simulink model "PMSM_FOC_Component_Baseline"  (R2025b)
settings: Solver=FixedStepDiscrete  StartTime=0.0  StopTime=4  FixedStep=0.0001  RelTol=1e-3
settings Model: Creator=Wu  LastModifiedBy=Wu
settings DataIOCC: SaveFormat=StructureWithTime  SignalLogging=off

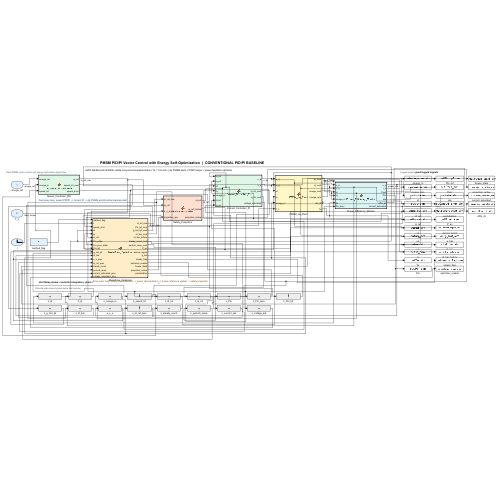
[thumbnail: Simulink's stored preview of the top-level diagram]
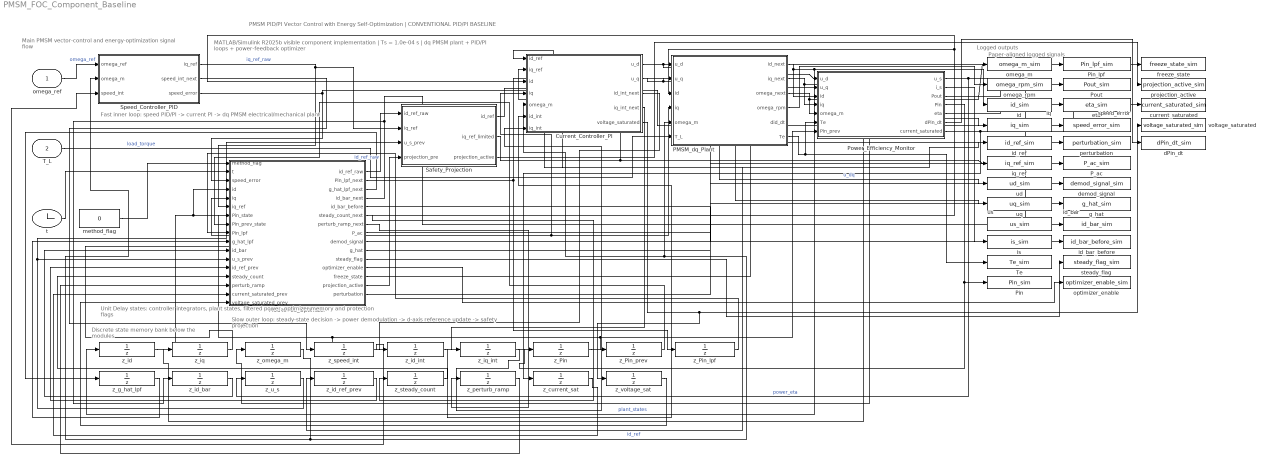
== system PMSM_FOC_Component_Baseline ==
  note: Main PMSM vector-control and energy-optimization signal flow
  note: Discrete state memory bank below the modules
  note: Logged outputs
  note: PMSM PID/PI Vector Control with Energy Self-Optimization | CONVENTIONAL PID/PI BASELINE
  note: MATLAB/Simulink R2025b visible component implementation | Ts = 1.0e-04 s | dq PMSM plant + PID/PI loops + power-feedback optimizer
  note: Fast inner loop: speed PID/PI -> current PI -> dq PMSM electrical/mechanical plant
  note: Slow outer loop: steady-state decision -> power demodulation -> d-axis reference update -> safety projection
  note: Unit Delay states: controller integrators, plant states, filtered power, optimizer memory and protection flags
  note: Paper-aligned logged signals
  omega_ref : Inport
  T_L : Inport  Port=2
  Current_Controller_PI : MATLAB Function  TreatAsAtomicUnit=on
  ModelFree_Optimizer : MATLAB Function  TreatAsAtomicUnit=on
  PMSM_dq_Plant : MATLAB Function  TreatAsAtomicUnit=on
  P_ac : ToWorkspace  VariableName=P_ac_sim  SaveFormat=Timeseries  SampleTime=-1
  Pin : ToWorkspace  VariableName=Pin_sim  SaveFormat=Timeseries  SampleTime=-1
  Pin_lpf : ToWorkspace  VariableName=Pin_lpf_sim  SaveFormat=Timeseries  SampleTime=-1
  Pout : ToWorkspace  VariableName=Pout_sim  SaveFormat=Timeseries  SampleTime=-1
  Power_Efficiency_Monitor : MATLAB Function  TreatAsAtomicUnit=on
  Safety_Projection : MATLAB Function  TreatAsAtomicUnit=on
  Speed_Controller_PID : MATLAB Function  TreatAsAtomicUnit=on
  Te : ToWorkspace  VariableName=Te_sim  SaveFormat=Timeseries  SampleTime=-1
  current_saturated : ToWorkspace  VariableName=current_saturated_sim  SaveFormat=Timeseries  SampleTime=-1
  dPin_dt : ToWorkspace  VariableName=dPin_dt_sim  SaveFormat=Timeseries  SampleTime=-1
  demod_signal : ToWorkspace  VariableName=demod_signal_sim  SaveFormat=Timeseries  SampleTime=-1
  eta : ToWorkspace  VariableName=eta_sim  SaveFormat=Timeseries  SampleTime=-1
  freeze_state : ToWorkspace  VariableName=freeze_state_sim  SaveFormat=Timeseries  SampleTime=-1
  g_hat : ToWorkspace  VariableName=g_hat_sim  SaveFormat=Timeseries  SampleTime=-1
  id : ToWorkspace  VariableName=id_sim  SaveFormat=Timeseries  SampleTime=-1
  id_bar : ToWorkspace  VariableName=id_bar_sim  SaveFormat=Timeseries  SampleTime=-1
  id_bar_before : ToWorkspace  VariableName=id_bar_before_sim  SaveFormat=Timeseries  SampleTime=-1
  id_ref : ToWorkspace  VariableName=id_ref_sim  SaveFormat=Timeseries  SampleTime=-1
  iq : ToWorkspace  VariableName=iq_sim  SaveFormat=Timeseries  SampleTime=-1
  iq_ref : ToWorkspace  VariableName=iq_ref_sim  SaveFormat=Timeseries  SampleTime=-1
  is : ToWorkspace  VariableName=is_sim  SaveFormat=Timeseries  SampleTime=-1
  method_flag : Constant  Value=0
  omega_m : ToWorkspace  VariableName=omega_m_sim  SaveFormat=Timeseries  SampleTime=-1
  omega_rpm : ToWorkspace  VariableName=omega_rpm_sim  SaveFormat=Timeseries  SampleTime=-1
  optimizer_enable : ToWorkspace  VariableName=optimizer_enable_sim  SaveFormat=Timeseries  SampleTime=-1
  perturbation : ToWorkspace  VariableName=perturbation_sim  SaveFormat=Timeseries  SampleTime=-1
  projection_active : ToWorkspace  VariableName=projection_active_sim  SaveFormat=Timeseries  SampleTime=-1
  speed_error : ToWorkspace  VariableName=speed_error_sim  SaveFormat=Timeseries  SampleTime=-1
  steady_flag : ToWorkspace  VariableName=steady_flag_sim  SaveFormat=Timeseries  SampleTime=-1
  t : Clock
  ud : ToWorkspace  VariableName=ud_sim  SaveFormat=Timeseries  SampleTime=-1
  uq : ToWorkspace  VariableName=uq_sim  SaveFormat=Timeseries  SampleTime=-1
  us : ToWorkspace  VariableName=us_sim  SaveFormat=Timeseries  SampleTime=-1
  voltage_saturated : ToWorkspace  VariableName=voltage_saturated_sim  SaveFormat=Timeseries  SampleTime=-1
  z_Pin : UnitDelay  SampleTime=0.0001  HasFrameUpgradeWarning=on
  z_Pin_lpf : UnitDelay  SampleTime=0.0001  HasFrameUpgradeWarning=on
  z_Pin_prev : UnitDelay  SampleTime=0.0001  HasFrameUpgradeWarning=on
  z_current_sat : UnitDelay  SampleTime=0.0001  HasFrameUpgradeWarning=on
  z_g_hat_lpf : UnitDelay  SampleTime=0.0001  HasFrameUpgradeWarning=on
  z_id : UnitDelay  SampleTime=0.0001  HasFrameUpgradeWarning=on
  z_id_bar : UnitDelay  SampleTime=0.0001  HasFrameUpgradeWarning=on
  z_id_int : UnitDelay  SampleTime=0.0001  HasFrameUpgradeWarning=on
  z_id_ref_prev : UnitDelay  SampleTime=0.0001  HasFrameUpgradeWarning=on
  z_iq : UnitDelay  SampleTime=0.0001  HasFrameUpgradeWarning=on
  z_iq_int : UnitDelay  SampleTime=0.0001  HasFrameUpgradeWarning=on
  z_omega_m : UnitDelay  SampleTime=0.0001  HasFrameUpgradeWarning=on
  z_perturb_ramp : UnitDelay  SampleTime=0.0001  HasFrameUpgradeWarning=on
  z_speed_int : UnitDelay  SampleTime=0.0001  HasFrameUpgradeWarning=on
  z_steady_count : UnitDelay  SampleTime=0.0001  HasFrameUpgradeWarning=on
  z_u_s : UnitDelay  SampleTime=0.0001  HasFrameUpgradeWarning=on
  z_voltage_sat : UnitDelay  SampleTime=0.0001  HasFrameUpgradeWarning=on
  wires:
  omega_ref/1 -> Speed_Controller_PID/1(omega_ref)  "omega_ref"
  z_omega_m/1 -> Speed_Controller_PID/2(omega_m), Current_Controller_PI/5(omega_m), PMSM_dq_Plant/5(omega_m)
  z_speed_int/1 -> Speed_Controller_PID/3(speed_int)
  method_flag/1 -> ModelFree_Optimizer/1(method_flag)
  t/1 -> ModelFree_Optimizer/2(t)
  Speed_Controller_PID/3(speed_error) -> speed_error/1, ModelFree_Optimizer/3(speed_error)
  z_id/1 -> Current_Controller_PI/3(id), PMSM_dq_Plant/3(id), ModelFree_Optimizer/4(id)
  z_iq/1 -> PMSM_dq_Plant/4(iq), Current_Controller_PI/4(iq), ModelFree_Optimizer/5(iq)
  Speed_Controller_PID/1(iq_ref) -> ModelFree_Optimizer/6(iq_ref), Safety_Projection/2(iq_ref)  "iq_ref_raw"
  z_Pin/1 -> ModelFree_Optimizer/7(Pin_state), z_Pin_prev/1, Power_Efficiency_Monitor/7(Pin_prev)
  z_Pin_prev/1 -> ModelFree_Optimizer/8(Pin_prev_state)
  z_Pin_lpf/1 -> ModelFree_Optimizer/9(Pin_lpf)
  z_g_hat_lpf/1 -> ModelFree_Optimizer/10(g_hat_lpf)
  z_id_bar/1 -> ModelFree_Optimizer/11(id_bar)
  z_u_s/1 -> ModelFree_Optimizer/12(u_s_prev), Safety_Projection/3(u_s_prev)
  z_id_ref_prev/1 -> ModelFree_Optimizer/13(id_ref_prev)
  z_steady_count/1 -> ModelFree_Optimizer/14(steady_count)
  z_perturb_ramp/1 -> ModelFree_Optimizer/15(perturb_ramp)
  z_current_sat/1 -> ModelFree_Optimizer/16(current_saturated_prev)
  z_voltage_sat/1 -> ModelFree_Optimizer/17(voltage_saturated_prev)
  ModelFree_Optimizer/1(id_ref_raw) -> Safety_Projection/1(id_ref_raw)  "id_ref_raw"
  ModelFree_Optimizer/14(projection_active) -> Safety_Projection/4(projection_pre)
  Safety_Projection/1(id_ref) -> id_ref/1, Current_Controller_PI/1(id_ref), z_id_ref_prev/1  "id_ref"
  Safety_Projection/2(iq_ref_limited) -> Current_Controller_PI/2(iq_ref), iq_ref/1
  z_id_int/1 -> Current_Controller_PI/6(id_int)
  z_iq_int/1 -> Current_Controller_PI/7(iq_int)
  Current_Controller_PI/1(u_d) -> Power_Efficiency_Monitor/1(u_d), ud/1, PMSM_dq_Plant/1(u_d)  "u_dq"
  Current_Controller_PI/2(u_q) -> Power_Efficiency_Monitor/2(u_q), uq/1, PMSM_dq_Plant/2(u_q)
  T_L/1 -> PMSM_dq_Plant/6(T_L)  "load_torque"
  PMSM_dq_Plant/1(id_next) -> id/1, z_id/1, Power_Efficiency_Monitor/3(id)  "plant_states"
  PMSM_dq_Plant/2(iq_next) -> iq/1, z_iq/1, Power_Efficiency_Monitor/4(iq)
  PMSM_dq_Plant/3(omega_next) -> omega_m/1, z_omega_m/1, Power_Efficiency_Monitor/5(omega_m)
  PMSM_dq_Plant/6(Te) -> Te/1, Power_Efficiency_Monitor/6(Te)
  Speed_Controller_PID/2(speed_int_next) -> z_speed_int/1
  Current_Controller_PI/3(id_int_next) -> z_id_int/1
  Current_Controller_PI/4(iq_int_next) -> z_iq_int/1
  Power_Efficiency_Monitor/4(Pin) -> z_Pin/1, Pin/1
  ModelFree_Optimizer/2(Pin_lpf_next) -> Pin_lpf/1, z_Pin_lpf/1
  ModelFree_Optimizer/3(g_hat_lpf_next) -> z_g_hat_lpf/1
  ModelFree_Optimizer/4(id_bar_next) -> id_bar/1, z_id_bar/1
  Power_Efficiency_Monitor/1(u_s) -> us/1, z_u_s/1  "power_eta"
  ModelFree_Optimizer/6(steady_count_next) -> z_steady_count/1
  ModelFree_Optimizer/7(perturb_ramp_next) -> z_perturb_ramp/1
  Power_Efficiency_Monitor/7(current_saturated) -> current_saturated/1, z_current_sat/1
  Current_Controller_PI/5(voltage_saturated) -> z_voltage_sat/1, voltage_saturated/1
  PMSM_dq_Plant/4(omega_rpm) -> omega_rpm/1
  Power_Efficiency_Monitor/2(i_s) -> is/1
  Power_Efficiency_Monitor/3(Pout) -> Pout/1
  Power_Efficiency_Monitor/5(eta) -> eta/1
  ModelFree_Optimizer/15(perturbation) -> perturbation/1
  ModelFree_Optimizer/8(P_ac) -> P_ac/1
  ModelFree_Optimizer/9(demod_signal) -> demod_signal/1
  ModelFree_Optimizer/10(g_hat) -> g_hat/1
  ModelFree_Optimizer/5(id_bar_before) -> id_bar_before/1
  ModelFree_Optimizer/11(steady_flag) -> steady_flag/1
  ModelFree_Optimizer/12(optimizer_enable) -> optimizer_enable/1
  ModelFree_Optimizer/13(freeze_state) -> freeze_state/1
  Safety_Projection/3(projection_active) -> projection_active/1
  Power_Efficiency_Monitor/6(dPin_dt) -> dPin_dt/1

== matlab function PMSM_FOC_Component_Baseline/PMSM_dq_Plant ==
  data: u_d input; id_next output; u_q input; id input; iq input; omega_m input; T_L input; iq_next output; omega_next output; omega_rpm output; did_dt output; Te output
function [id_next, iq_next, omega_next, omega_rpm, did_dt, Te] = PMSM_dq_Plant(u_d, u_q, id, iq, omega_m, T_L)
%#codegen
Ts=0.0001; polePairs=4; Rs=0.80000000000000004; Ld=0.0035000000000000001; Lq=0.0085000000000000006; psi=0.105; J=0.002; B=0.00050000000000000001;
omega_e = polePairs * omega_m;
did_dt = (u_d - Rs * id + omega_e * Lq * iq) / Ld;
diq_dt = (u_q - Rs * iq - omega_e * (Ld * id + psi)) / Lq;
Te = 1.5 * polePairs * (psi * iq + (Ld - Lq) * id * iq);
domega_dt = (Te - T_L - B * omega_m) / J;
id_next = id + Ts * did_dt;
iq_next = iq + Ts * diq_dt;
omega_next = max(0, omega_m + Ts * domega_dt);
omega_rpm = omega_next * 60 / (2*pi);
end

== matlab function PMSM_FOC_Component_Baseline/Power_Efficiency_Monitor ==
  data: u_d input; u_s output; u_q input; id input; iq input; omega_m input; Te input; Pin_prev input; i_s output; Pout output; Pin output; eta output; dPin_dt output; current_saturated output
function [u_s, i_s, Pout, Pin, eta, dPin_dt, current_saturated] = Power_Efficiency_Monitor(u_d, u_q, id, iq, omega_m, Te, Pin_prev)
%#codegen
Ts=0.0001; Imax=25;
u_s = hypot(u_d, u_q);
i_s = hypot(id, iq);
Pin = 1.5 * (u_d * id + u_q * iq);
Pout = max(0, Te * omega_m);
eta = 0;
if Pin > 1e-9
    eta = min(max(Pout / Pin, 0), 1.2);
end
dPin_dt = (Pin - Pin_prev) / max(Ts, eps);
current_saturated = double(i_s > Imax * 0.999);
end

== matlab function PMSM_FOC_Component_Baseline/ModelFree_Optimizer ==
  data: method_flag input; id_ref_raw output; t input; speed_error input; id input; iq input; iq_ref input; Pin_state input; Pin_prev_state input; Pin_lpf input; g_hat_lpf input; id_bar input; u_s_prev input; id_ref_prev input; steady_count input; perturb_ramp input; current_saturated_prev input; voltage_saturated_prev input; Pin_lpf_next output; g_hat_lpf_next output; id_bar_next output; id_bar_before output; steady_count_next output; perturb_ramp_next output; P_ac output; demod_signal output; g_hat output; steady_flag output; optimizer_enable output; freeze_state output; projection_active output; perturbation output
function [id_ref_raw, Pin_lpf_next, g_hat_lpf_next, id_bar_next, id_bar_before, steady_count_next, perturb_ramp_next, P_ac, demod_signal, g_hat, steady_flag, optimizer_enable, freeze_state, projection_active, perturbation] = ModelFree_Optimizer(method_flag, t, speed_error, id, iq, iq_ref, Pin_state, Pin_prev_state, Pin_lpf, g_hat_lpf, id_bar, u_s_prev, id_ref_prev, steady_count, perturb_ramp, current_saturated_prev, voltage_saturated_prev)
%#codegen
Ts=0.0001; omegaErrTh=5; idErrTh=0.5; iqErrTh=0.5; powerSlopeTh=1000000; holdTime=0.41999999999999998;
amp=0.10000000000000001; omegaD=37.699111843077517; pinTau=0.059999999999999998; gradTau=0.10000000000000001; alpha=10; updatePeriod=0.0001; maxStep=0.002; rateLimit=25; resumeRamp=0.050000000000000003; freezeRamp=0.080000000000000002;
searchBiasRate=0; searchBiasTau=1; searchBiasStopId=-Inf;
Imax=25; idMin=-18; idMax=4; Vmax=173.20508075688775; vProjStep=0.02;
id_bar_before = id_bar;
P_ac = Pin_state - Pin_lpf;
demod_signal = 0;
g_hat = g_hat_lpf;
steady_flag = 0;
optimizer_enable = 0;
projection_active = 0;
freeze_state = 1;
perturbation = 0;
Pin_lpf_next = Pin_lpf;
g_hat_lpf_next = g_hat_lpf;
id_bar_next = id_bar;
steady_count_next = steady_count;
perturb_ramp_next = perturb_ramp;
if method_flag > 0.5
    dPin_dt = (Pin_state - Pin_prev_state) / max(Ts, eps);
    cond_speed = abs(speed_error) < omegaErrTh;
    cond_id = abs(id_ref_prev - id) < idErrTh;
    cond_iq = abs(iq_ref - iq) < iqErrTh;
    cond_power = abs(dPin_dt) < powerSlopeTh;
    cond_sat = ~(current_saturated_prev > 0.5 || voltage_saturated_prev > 0.5);
    if cond_speed && cond_id && cond_iq && cond_power && cond_sat
        steady_count_next = steady_count + 1;
    else
        steady_count_next = 0;
    end
    steady_flag = double(steady_count_next * Ts >= holdTime);
    beta_pin = Ts / (pinTau + Ts);
    beta_grad = Ts / (gradTau + Ts);
    Pin_lpf_next = Pin_lpf + beta_pin * (Pin_state - Pin_lpf);
    P_ac = Pin_state - Pin_lpf_next;
    sin_d = sin(omegaD * t);
    demod_signal = P_ac * sin_d;
    g_hat_lpf_next = g_hat_lpf + beta_grad * (demod_signal - g_hat_lpf);
    g_hat = 2 * g_hat_lpf_next / max(amp, eps);
    if steady_flag > 0.5
        optimizer_enable = 1;
        freeze_state = 0;
        update = clamp(-alpha * g_hat * updatePeriod, -maxStep, maxStep);
        if searchBiasRate > 0 && id_bar > searchBiasStopId
            biasAge = max(t - holdTime, 0);
            biasRamp = 1 - exp(-biasAge / max(searchBiasTau, Ts));
            update = update + searchBiasRate * biasRamp * (searchBiasStopId - id_bar) * Ts;
        end
        id_bar_candidate = id_bar + update;
        [id_bar_projected, projection_active] = project_id_reference(id_bar_candidate, iq_ref, u_s_prev, Imax, idMin, idMax, Vmax, vProjStep);
        id_bar_next = slew_limit(id_bar_projected, id_bar, rateLimit, Ts);
        perturb_ramp_next = min(1, perturb_ramp + Ts / max(resumeRamp, Ts));
        perturbation = perturb_ramp_next * amp * sin_d;
    else
        perturb_ramp_next = max(0, perturb_ramp - Ts / max(freezeRamp, Ts));
        perturbation = perturb_ramp_next * amp * sin(omegaD * t);
    end
    id_ref_raw = id_bar_next + perturbation;
else
    id_ref_raw = 0;
end
end

function [id_projected, active] = project_id_reference(id_candidate, iq_ref, u_s_est, Imax, idMin, idMax, Vmax, vProjStep)
id_projected = clamp(id_candidate, idMin, idMax);
box_active = abs(id_projected - id_candidate) > 1e-12;
id_limit = sqrt(max(Imax^2 - iq_ref^2, 0));
id_after_current = clamp(id_projected, -id_limit, id_limit);
current_active = abs(id_after_current - id_projected) > 1e-12;
id_projected = clamp(id_after_current, idMin, idMax);
voltage_active = u_s_est > Vmax * 0.995;
if voltage_active
    id_projected = max(idMin, id_projected - vProjStep);
end
id_projected = clamp(id_projected, idMin, idMax);
active = double(box_active || current_active || voltage_active);
end

function y = slew_limit(target, current, rate, Ts)
delta = clamp(target - current, -rate * Ts, rate * Ts);
y = current + delta;
end

function y = clamp(x, lo, hi)
y = min(max(x, lo), hi);
end

== matlab function PMSM_FOC_Component_Baseline/Speed_Controller_PID ==
  data: omega_ref input; iq_ref output; omega_m input; speed_int input; speed_int_next output; speed_error output
function [iq_ref, speed_int_next, speed_error] = Speed_Controller_PID(omega_ref, omega_m, speed_int)
%#codegen
Ts = 0.0001; Kp = 0.16; Ki = 7; Imax = 25; intLimit = 80;
speed_error = omega_ref - omega_m;
speed_int_next = clamp(speed_int + speed_error * Ts, -intLimit, intLimit);
iq_raw = Kp * speed_error + Ki * speed_int_next;
iq_ref = clamp(iq_raw, -Imax, Imax);
if abs(iq_ref - iq_raw) > 1e-12 && sign(speed_error) == sign(iq_raw)
    speed_int_next = speed_int;
end
end

function y = clamp(x, lo, hi)
y = min(max(x, lo), hi);
end

== matlab function PMSM_FOC_Component_Baseline/Safety_Projection ==
  data: id_ref_raw input; id_ref output; iq_ref input; u_s_prev input; projection_pre input; iq_ref_limited output; projection_active output
function [id_ref, iq_ref_limited, projection_active] = Safety_Projection(id_ref_raw, iq_ref, u_s_prev, projection_pre)
%#codegen
Imax=25; idMin=-18; idMax=4; Vmax=173.20508075688775; vProjStep=0.02;
[id_ref, proj_final] = project_id_reference(id_ref_raw, iq_ref, u_s_prev, Imax, idMin, idMax, Vmax, vProjStep);
iq_limit = sqrt(max(Imax^2 - id_ref^2, 0));
iq_ref_limited = clamp(iq_ref, -iq_limit, iq_limit);
projection_active = double(projection_pre > 0.5 || proj_final > 0.5);
end

function [id_projected, active] = project_id_reference(id_candidate, iq_ref, u_s_est, Imax, idMin, idMax, Vmax, vProjStep)
id_projected = clamp(id_candidate, idMin, idMax);
box_active = abs(id_projected - id_candidate) > 1e-12;
id_limit = sqrt(max(Imax^2 - iq_ref^2, 0));
id_after_current = clamp(id_projected, -id_limit, id_limit);
current_active = abs(id_after_current - id_projected) > 1e-12;
id_projected = clamp(id_after_current, idMin, idMax);
voltage_active = u_s_est > Vmax * 0.995;
if voltage_active
    id_projected = max(idMin, id_projected - vProjStep);
end
id_projected = clamp(id_projected, idMin, idMax);
active = double(box_active || current_active || voltage_active);
end

function y = clamp(x, lo, hi)
y = min(max(x, lo), hi);
end

== matlab function PMSM_FOC_Component_Baseline/Current_Controller_PI ==
  data: id_ref input; u_d output; iq_ref input; id input; iq input; omega_m input; id_int input; iq_int input; u_q output; id_int_next output; iq_int_next output; voltage_saturated output
function [u_d, u_q, id_int_next, iq_int_next, voltage_saturated] = Current_Controller_PI(id_ref, iq_ref, id, iq, omega_m, id_int, iq_int)
%#codegen
Ts=0.0001; polePairs=4; Ld=0.0035000000000000001; Lq=0.0085000000000000006; psi=0.105; Vmax=173.20508075688775;
Kpd=4.2000000000000002; Kid=850; Kpq=8.5; Kiq=850; intLimit=120;
omega_e = polePairs * omega_m;
e_d = id_ref - id;
e_q = iq_ref - iq;
id_int_try = id_int + e_d * Ts;
iq_int_try = iq_int + e_q * Ts;
u_d_raw = Kpd * e_d + Kid * id_int_try - omega_e * Lq * iq;
u_q_raw = Kpq * e_q + Kiq * iq_int_try + omega_e * (Ld * id + psi);
u_raw = hypot(u_d_raw, u_q_raw);
voltage_saturated = double(u_raw > Vmax);
if voltage_saturated > 0.5
    scale = Vmax / max(u_raw, eps);
    u_d = u_d_raw * scale;
    u_q = u_q_raw * scale;
    id_int_next = id_int;
    iq_int_next = iq_int;
else
    u_d = u_d_raw;
    u_q = u_q_raw;
    id_int_next = clamp(id_int_try, -intLimit, intLimit);
    iq_int_next = clamp(iq_int_try, -intLimit, intLimit);
end
end

function y = clamp(x, lo, hi)
y = min(max(x, lo), hi);
end
